simulink model "b3"  (R2020a)
settings: Solver=VariableStepAuto  StartTime=0.0  StopTime=10.0  RelTol=1e-3
libraries: simulink x1
settings Model: Creator=Erfan  LastModifiedBy=Erfan

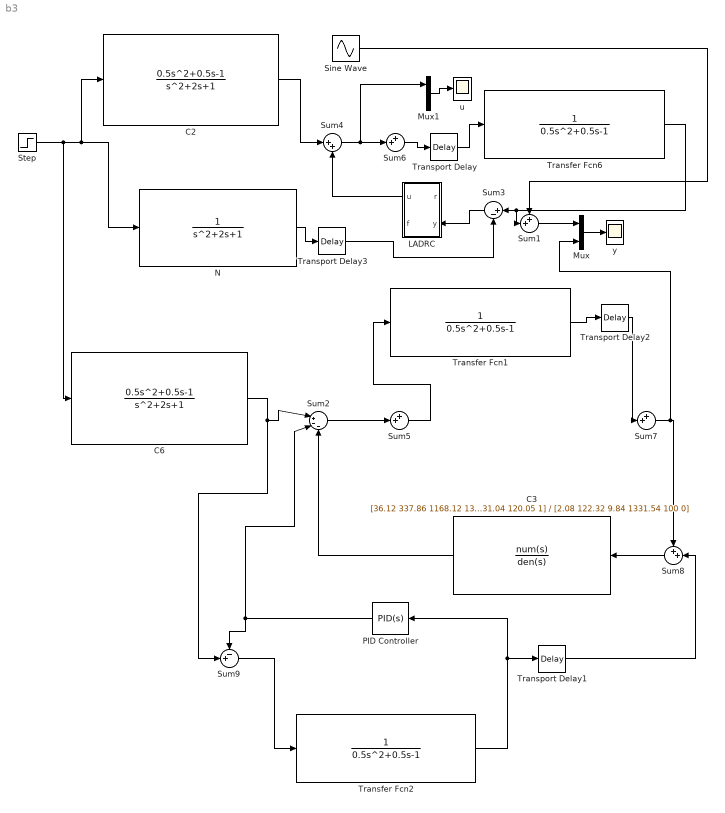
== system b3 ==
  C2 : TransferFcn  Numerator=[0.5 0.5 -1]
  C3 : TransferFcn  Numerator=[36.12 337.86 1168.12 1331.04 120.05 1]  Denominator=[2.08 122.32 9.84 1331.54 100 0]
  C6 : TransferFcn  Numerator=[0.5 0.5 -1]
  LADRC : Subsystem  mask{n=4, b0=1, Ko=[106.3492 212.5218 164.8019 14.6933 1], Lo=[102.7067 3422.9873 -4854.4554 5294.1912 66.4426]'}
      mask prompts: n "order"; b0 "high-frequency gain"; Ko "feedback gain"; Lo "observer gain"
  Mux : Mux  Inputs=2
  Mux1 : Mux  Inputs=2
  N : TransferFcn  Numerator=1
  PID Controller : simulink/Continuous/PID Controller  Controller=PID  Form=Parallel  TimeDomain=Continuous-time  UseExternalTs=off  SampleTime=1  IntegratorMethod=Forward Euler  FilterMethod=Forward Euler  ControllerParametersSource=internal  P=11.7545892549716  I=6.76343430748452  D=4.31400914921107  UseFilter=on  N=24.1500506670773  TunerSelectOption=Transfer Function Based (PID Tuner App)  InitialConditionSource=internal  InitialConditionForIntegrator=0  InitialConditionForFilter=0  DifferentiatorICPrevScaledInput=0  ExternalReset=none  TrackingMode=off  Kt=1  LimitOutput=off  UpperSaturationLimit=inf  LowerSaturationLimit=-inf  LinearizeAsGain=on  AntiWindupMode=none  Kb=1  POutMin=[]  POutMax=[]  IOutMin=[]  IOutMax=[]  DOutMin=[]  DOutMax=[]  NOutMin=[]  NOutMax=[]  SumOutMin=[]  SumOutMax=[]  SaturationOutMin=[]  SaturationOutMax=[]  PParamMin=[]  PParamMax=[]  IParamMin=[]  IParamMax=[]  DParamMin=[]  DParamMax=[]  NParamMin=[]  NParamMax=[]  KbParamMin=[]  KbParamMax=[]  KtParamMin=[]  KtParamMax=[]  KbOutMin=[]  KbOutMax=[]  KtOutMin=[]  KtOutMax=[]  IntegratorOutMin=[]  IntegratorOutMax=[]  FilterOutMin=[]  FilterOutMax=[]  SumI1OutMin=[]  SumI1OutMax=[]  SumI2OutMin=[]  SumI2OutMax=[]  SumI3OutMin=[]  SumI3OutMax=[]  SumI4OutMin=[]  SumI4OutMax=[]  SumDOutMin=[]  SumDOutMax=[]  DifferentiatorOutMin=[]  DifferentiatorOutMax=[]  FilterDiffOutCoefMin=[]  FilterDiffOutCoefMax=[]  ReciprocalOutMin=[]  ReciprocalOutMax=[]  SumDenOutMin=[]  SumDenOutMax=[]  SumNumOutMin=[]  SumNumOutMax=[]  DivideOutMin=[]  DivideOutMax=[]  UdiffTsProdOutMin=[]  UdiffTsProdOutMax=[]  NTsProdOutMin=[]  NTsProdOutMax=[]  UintegralTsProdOutMin=[]  UintegralTsProdOutMax=[]  UngainTsProdOutMin=[]  UngainTsProdOutMax=[]  IntegratorContinuousStateAttributes=''  IntegratorStateMustResolveToSignalObject=off  IntegratorRTWStateStorageClass=Auto  FilterContinuousStateAttributes=''  FilterStateMustResolveToSignalObject=off  FilterRTWStateStorageClass=Auto  ParallelPVariant=InternalParameters  IdealPVariant=Disabled  IVariant=InternalParameters  DVariant=InternalParameters  IntegratorVariant=Continuous  SatVariant=Disabled  AWVariant=Passthrough  PCopyVariant=Disabled  TRVariant=Disabled  FdbkBlocksVariant=Forward  IdealPFdbkVariant=Disabled  SatFdbkVariant=Disabled  DerivativeFilterVariant=ContFilter  NVariant=InternalParameters  NCopyVariant=Disabled  FilterICVariant=InternalICsFilter  IntegratorICVariant=InternalICs  ExternalResetVariant=Disabled  TRSumVariant=Passthrough  SumFdbkVariant=Disabled  SumVariant=Sum_PID  TsampFilterVariant=InternalTs  TsampNgainVariant=Passthrough  TsampIntegralVariant=Passthrough
  Sine Wave : Sin  Amplitude=0.02  SampleTime=0
  Step : Step  Time=0  SampleTime=0
  Sum{1,5..8} (5 alike) : Sum  Inputs=++|  InputSameDT=on  SaturateOnIntegerOverflow=on  OutDataTypeStr=Inherit: Same as first input
  Sum2 : Sum  Inputs=|+--  SaturateOnIntegerOverflow=on
  Sum3 : Sum  Inputs=|+-  SaturateOnIntegerOverflow=on
  Sum4 : Sum  Inputs=|++  SaturateOnIntegerOverflow=on
  Sum9 : Sum  Inputs=-+|  InputSameDT=on  SaturateOnIntegerOverflow=on  OutDataTypeStr=Inherit: Same as first input
  Transfer Fcn1 : TransferFcn  Numerator=1  Denominator=[0.5 0.5 -1]
  Transfer Fcn2 : TransferFcn  Numerator=1  Denominator=[0.5 0.5 -1]
  Transfer Fcn6 : TransferFcn  Numerator=1  Denominator=[0.5 0.5 -1]
  Transport Delay{,1..3} (4 alike) : TransportDelay  DelayTime=1.2
  u : Scope
  y : Scope
  wires:
  Transport Delay3/1 -> Sum3/2
  Sum6/1 -> Transport Delay/1
  Sum2/1 -> Sum5/2
  Transport Delay/1 -> Transfer Fcn6/1
  Sum4/1 -> Mux1/1, Sum6/2
  LADRC/1(u) -> Sum4/2
  Mux/1 -> y/1
  C2/1 -> Sum4/1
  Sum7/1 -> Mux/2, Sum8/1
  Transfer Fcn1/1 -> Transport Delay2/1
  Step/1 -> C6/1, N/1, C2/1
  Sum9/1 -> Transfer Fcn2/1
  Transfer Fcn2/1 -> PID Controller/1, Transport Delay1/1
  Sum8/1 -> C3/1
  Sum3/1 -> LADRC/2(y)
  Sum5/1 -> Transfer Fcn1/1
  C6/1 -> Sum9/2, Sum2/1
  N/1 -> Transport Delay3/1
  Sine Wave/1 -> Sum1/1
  Sum1/1 -> Mux/1
  C3/1 -> Sum2/3
  PID Controller/1 -> Sum9/1, Sum2/2
  Transfer Fcn6/1 -> Sum1/2, Sum3/1
  Transport Delay2/1 -> Sum7/2
  Transport Delay1/1 -> Sum8/2
  Mux1/1 -> u/1

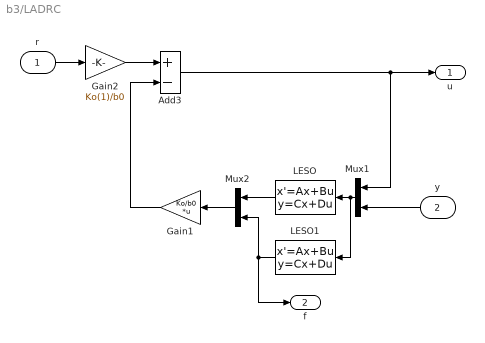
== system b3/LADRC ==
  r : Inport
  y : Inport  Port=2
  Add3 : Sum  Inputs=+-
  Gain1 : Gain  Gain=Ko/b0  Multiplication=Matrix(K*u)
  Gain2 : Gain  Gain=Ko(1)/b0
  LESO : StateSpace  A=[zeros(n,1) eye(n,n);zeros(1,n+1)]-Lo*[1 zeros(1,n)]  B=[[zeros(n-1,1);b0;0] Lo]  C=[eye(n,n) zeros(n,1)]  D=zeros(n,2)  InitialCondition=0
  LESO1 : StateSpace  A=[zeros(n,1) eye(n,n);zeros(1,n+1)]-Lo*[1 zeros(1,n)]  B=[[zeros(n-1,1);b0;0] Lo]  C=[zeros(1,n) 1]  D=[0 0]  InitialCondition=0
  Mux1 : Mux  Inputs=2
  Mux2 : Mux  Inputs=2
  u : Outport
  f : Outport  Port=2
  wires:
  Gain1/1 -> Add3/2
  LESO1/1 -> Mux2/2, f/1
  Mux2/1 -> Gain1/1
  LESO/1 -> Mux2/1
  r/1 -> Gain2/1
  Mux1/1 -> LESO/1, LESO1/1
  y/1 -> Mux1/2
  Add3/1 -> Mux1/1, u/1
  Gain2/1 -> Add3/1
